simulink model "car_longitudinal_dynamics_plant"  (R2024b)
settings: Solver=ode45  StartTime=0.0  StopTime=10.0  RelTol=1e-3
values from neighbouring files (symbols this model uses):
  airDensityKgpm3 = 1.225    [initial.m]
  areaM2 = 2.5    [initial.m]
  coeffDrag = 0.28    [initial.m]
  gravityMps2 = 9.81    [initial.m]
  massKg = 2500    [initial.m]
  massKg1 = 2400    [initial.m]
  mu = 0.7    [constraint.m]    (also in initial.m; objective.m; sfunction_sid.m)
settings Model: Creator=EWiputr  LastModifiedBy=siddhik
settings SolverCC: ZeroCrossAlgorithm=Adaptive
settings OptimizationCC: ReuseModelBlockBuffer=off
settings DebuggingCC: IgnoredZcDiagnostic=none
settings RTWCC: GPUComputeCapability=3.5

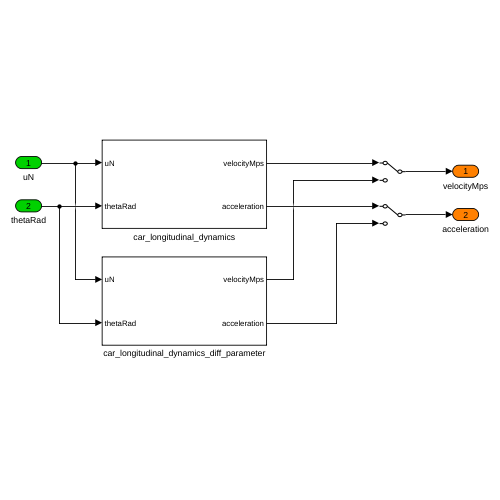
[thumbnail: Simulink's stored preview of the top-level diagram]
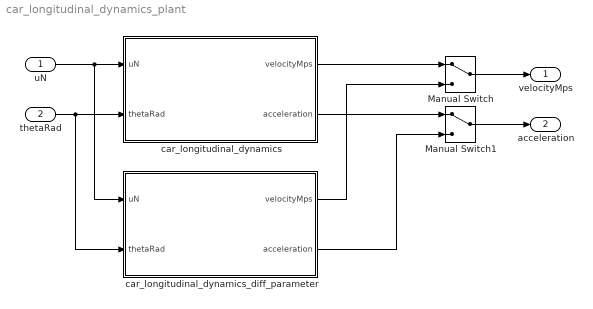
== system car_longitudinal_dynamics_plant ==
  uN : Inport
  thetaRad : Inport  Port=2
  Manual Switch : ManualSwitch
  Manual Switch1 : ManualSwitch
  car_longitudinal_dynamics : Subsystem
  car_longitudinal_dynamics_diff_parameter : Subsystem
  velocityMps : Outport
  acceleration : Outport  Port=2
  wires:
  uN/1 -> car_longitudinal_dynamics_diff_parameter/1(uN), car_longitudinal_dynamics/1(uN)
  thetaRad/1 -> car_longitudinal_dynamics/2(thetaRad), car_longitudinal_dynamics_diff_parameter/2(thetaRad)
  car_longitudinal_dynamics_diff_parameter/1(velocityMps) -> Manual Switch/2
  Manual Switch/1 -> velocityMps/1
  car_longitudinal_dynamics/1(velocityMps) -> Manual Switch/1
  Manual Switch1/1 -> acceleration/1
  car_longitudinal_dynamics/2(acceleration) -> Manual Switch1/1
  car_longitudinal_dynamics_diff_parameter/2(acceleration) -> Manual Switch1/2

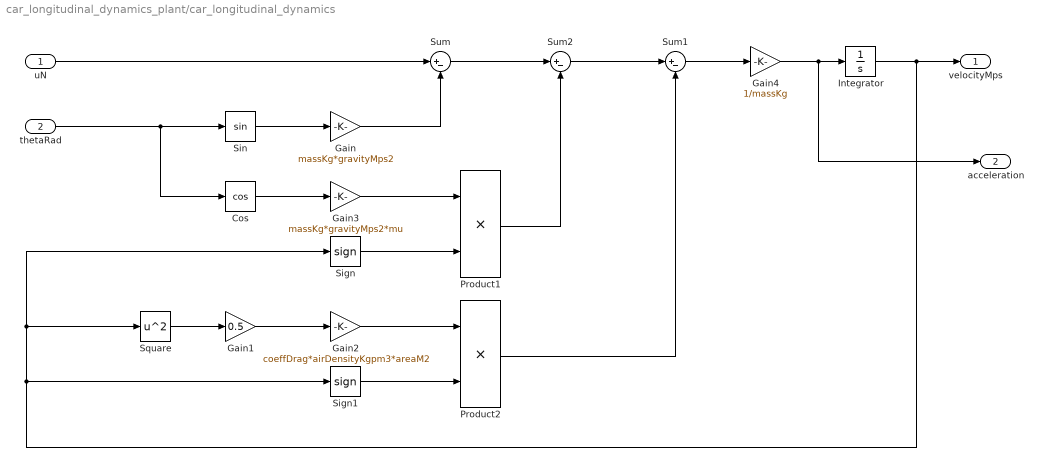
== system car_longitudinal_dynamics_plant/car_longitudinal_dynamics ==
  uN : Inport
  thetaRad : Inport  Port=2
  Cos : Trigonometry  Operator=cos
  Gain : Gain  Gain=massKg*gravityMps2
      settings: AttributesFormatString=%<Gain>
  Gain1 : Gain  Gain=0.5
      settings: AttributesFormatString=%<Gain>
  Gain2 : Gain  Gain=coeffDrag*airDensityKgpm3*areaM2
      settings: AttributesFormatString=%<Gain>
  Gain3 : Gain  Gain=massKg*gravityMps2*mu
      settings: AttributesFormatString=%<Gain>
  Gain4 : Gain  Gain=1/massKg
      settings: AttributesFormatString=%<Gain>
  Integrator : Integrator
  Product1 : Product
  Product2 : Product
  Sign : Signum
  Sign1 : Signum
  Sin : Trigonometry
  Square : Math  Operator=square
  Sum : Sum  Inputs=|+-
  Sum1 : Sum  Inputs=|+-
  Sum2 : Sum  Inputs=|+-
  velocityMps : Outport
  acceleration : Outport  Port=2
  wires:
  uN/1 -> Sum/1
  thetaRad/1 -> Sin/1, Cos/1
  Gain1/1 -> Gain2/1
  Gain2/1 -> Product2/1
  Integrator/1 -> velocityMps/1, Sign1/1, Sign/1, Square/1
  Product2/1 -> Sum1/2
  Sum2/1 -> Sum1/1
  Sum/1 -> Sum2/1
  Sin/1 -> Gain/1
  Gain/1 -> Sum/2
  Cos/1 -> Gain3/1
  Gain3/1 -> Product1/1
  Product1/1 -> Sum2/2
  Sum1/1 -> Gain4/1
  Gain4/1 -> acceleration/1, Integrator/1
  Square/1 -> Gain1/1
  Sign/1 -> Product1/2
  Sign1/1 -> Product2/2

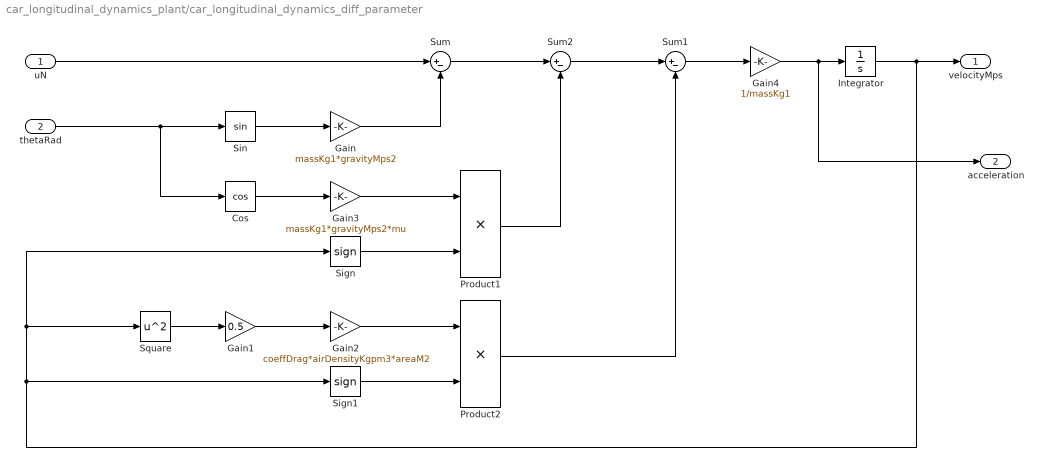
== system car_longitudinal_dynamics_plant/car_longitudinal_dynamics_diff_parameter ==
  uN : Inport
  thetaRad : Inport  Port=2
  Cos : Trigonometry  Operator=cos
  Gain : Gain  Gain=massKg1*gravityMps2
      settings: AttributesFormatString=%<Gain>
  Gain1 : Gain  Gain=0.5
      settings: AttributesFormatString=%<Gain>
  Gain2 : Gain  Gain=coeffDrag*airDensityKgpm3*areaM2
      settings: AttributesFormatString=%<Gain>
  Gain3 : Gain  Gain=massKg1*gravityMps2*mu
      settings: AttributesFormatString=%<Gain>
  Gain4 : Gain  Gain=1/massKg1
      settings: AttributesFormatString=%<Gain>
  Integrator : Integrator
  Product1 : Product
  Product2 : Product
  Sign : Signum
  Sign1 : Signum
  Sin : Trigonometry
  Square : Math  Operator=square
  Sum : Sum  Inputs=|+-
  Sum1 : Sum  Inputs=|+-
  Sum2 : Sum  Inputs=|+-
  velocityMps : Outport
  acceleration : Outport  Port=2
  wires:
  uN/1 -> Sum/1
  thetaRad/1 -> Sin/1, Cos/1
  Gain1/1 -> Gain2/1
  Gain2/1 -> Product2/1
  Integrator/1 -> velocityMps/1, Sign1/1, Sign/1, Square/1
  Product2/1 -> Sum1/2
  Sum2/1 -> Sum1/1
  Sum/1 -> Sum2/1
  Sin/1 -> Gain/1
  Gain/1 -> Sum/2
  Cos/1 -> Gain3/1
  Gain3/1 -> Product1/1
  Product1/1 -> Sum2/2
  Sum1/1 -> Gain4/1
  Gain4/1 -> acceleration/1, Integrator/1
  Square/1 -> Gain1/1
  Sign/1 -> Product1/2
  Sign1/1 -> Product2/2
